simulink model "robot_arm_pi2"  (R2024a)
settings: Solver=VariableStepAuto  StartTime=0.0  StopTime=Tsim  RelTol=1e-3
values from neighbouring files (symbols this model uses):
  mag = 0.1    [one_link_robot_arm_integral.m]    (also in robot_arm_pi.m = 1; robot_arm_state_feedback.m = 1; robust_state_feedback.m = 1)
  Ts = 0.1    [one_link_robot_arm_integral.m]    (also in robot_arm_pi.m; robot_arm_state_feedback.m)
  x0 = (2*mx0).*rand(5,1)-mx0    [one_link_robot_arm_integral.m]    (also in robot_arm_pi.m = (2*mag).*rand(5,1)-mag; robot_arm_state_feedback.m = (2*mag).*rand(n,1)-mag)
settings Model: Creator=pietrotesi  LastModifiedBy=watch
settings SolverCC: AlgebraicLoopSolver=TrustRegion
settings DataIOCC: ReturnWorkspaceOutputs=off
settings DebuggingCC: UnconnectedInputMsg=warning  UnconnectedOutputMsg=warning  UnconnectedLineMsg=warning
settings ModelReferenceCC: EnableRefExpFcnMdlSchedulingChecks=on
settings RTWCC: GPUComputeCapability=3.5  DLArmComputeVersion=19.05

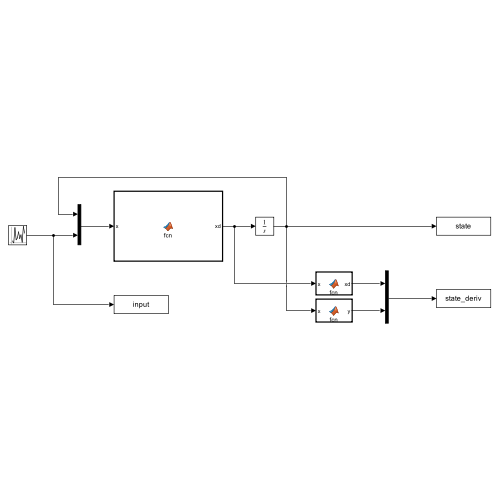
[thumbnail: Simulink's stored preview of the top-level diagram]
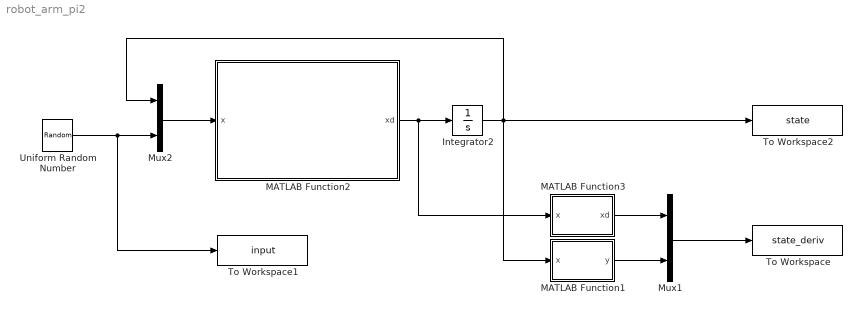
== system robot_arm_pi2 ==
  Integrator2 : Integrator  InitialCondition=x0
  MATLAB Function1 : MATLAB Function  TreatAsAtomicUnit=on
  MATLAB Function2 : MATLAB Function  TreatAsAtomicUnit=on
  MATLAB Function3 : MATLAB Function  TreatAsAtomicUnit=on
  Mux1 : Mux  Inputs=2
  Mux2 : Mux  Inputs=2
  To Workspace : ToWorkspace  VariableName=state_deriv  SaveFormat=Structure With Time  SampleTime=Ts
  To Workspace1 : ToWorkspace  VariableName=input  SaveFormat=Structure With Time  SampleTime=Ts
  To Workspace2 : ToWorkspace  VariableName=state  SaveFormat=Structure With Time  SampleTime=Ts
  Uniform Random Number : UniformRandomNumber  Minimum=-mag  Maximum=mag  SampleTime=Ts
  wires:
  Mux2/1 -> MATLAB Function2/1(x)
  MATLAB Function2/1(xd) -> MATLAB Function3/1(x), Integrator2/1
  Uniform Random Number/1 -> To Workspace1/1, Mux2/2
  Integrator2/1 -> To Workspace2/1, MATLAB Function1/1(x), Mux2/1
  Mux1/1 -> To Workspace/1
  MATLAB Function1/1(y) -> Mux1/2
  MATLAB Function3/1(xd) -> Mux1/1

== matlab function robot_arm_pi2/MATLAB Function2 ==
  data: x input; xd output
function xd = fcn(x)
target = pi/3; % Track reference
noise = [0.1 0.2 0.3 0.4]';
x1 = x(1);
u  = x(6);

A = [0 1 0 0; ... % precomputed A matrix
    -2 -0.75 1 0; ...
    0 0 0 1; ...
    -1.3 0 0.66 -0.2];
B = [0; 0; 0; 6.6]; % precomputed B matrix
% noise = 0.1 * (2*rand(4,1) - 1);

xd = [A*x(1:4) + B*u + noise; x1 - target];

== matlab function robot_arm_pi2/MATLAB Function3 ==
  data: x input; xd output
function xd = fcn(x)

xd = x(1:4,1);

== matlab function robot_arm_pi2/MATLAB Function1 ==
  data: x input; y output
function y = fcn(x)

y = x(1);
